simulink model "TopModel"  (R2019b)
settings: Solver=VariableStepAuto  StartTime=0.0  StopTime=10  RelTol=1e-3
model workspace (MAT data in the model file):
  J = 0.02
  Kb = 0.1
  Kf = 0.2
  Km = 0.1
  L = 0.5
  R = 2
  ctrlDen = [1 0]
  ctrlNum = [2.02136445733 8.39446937163]
settings Model: OrderedModelArguments=off  Creator=cleme  LastModifiedBy=cleme
settings DataIOCC: ReturnWorkspaceOutputs=off
settings DebuggingCC: ArithmeticOperatorsInVariantConditions=warning
settings SFSimCC: CustomCodeUndefinedFunction=UseInterfaceOnly

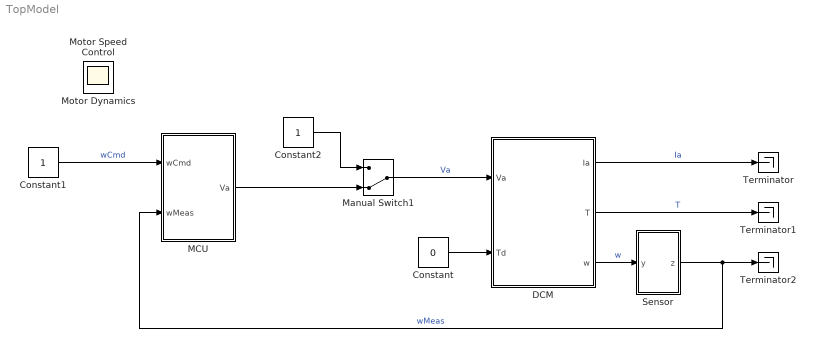
== system TopModel ==
  Constant : Constant  Value=0
  Constant1 : Constant
  Constant2 : Constant
  DCM : Subsystem
  MCU : Subsystem
  Manual Switch1 : ManualSwitch  CurrentSetting=0
  Sensor : Subsystem
  Terminator : Terminator
  Terminator1 : Terminator
  Terminator2 : Terminator
  Motor Dynamics : Scope
  Motor Speed Control : Scope
  wires:
  Constant/1 -> DCM/2(Td)
  Sensor/1(z) -> MCU/2(wMeas), Terminator2/1  "wMeas"
  DCM/3(w) -> Sensor/1(y)  "w"
  Manual Switch1/1 -> DCM/1(Va)  "Va"
  DCM/1(Ia) -> Terminator/1  "Ia"
  DCM/2(T) -> Terminator1/1  "T"
  Constant2/1 -> Manual Switch1/1
  Constant1/1 -> MCU/1(wCmd)  "wCmd"
  MCU/1(Va) -> Manual Switch1/2

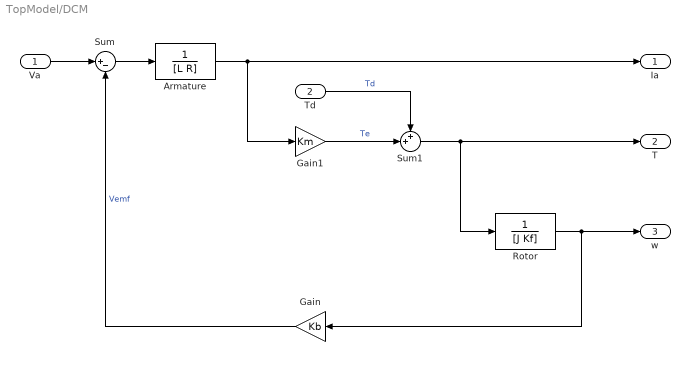
== system TopModel/DCM ==
  Va : Inport  Unit=V
  Td : Inport  Port=2  Unit=N*m
  Armature : TransferFcn  Numerator=1  Denominator=[L R]
  Gain : Gain  Gain=Kb
  Gain1 : Gain  Gain=Km
  Rotor : TransferFcn  Denominator=[J Kf]
  Sum : Sum  Inputs=|+-
  Sum1 : Sum  Inputs=++|
  Ia : Outport
  T : Outport  Port=2
  w : Outport  Port=3  Unit=rad/s  VectorParamsAs1DForOutWhenUnconnected=off
  wires:
  Sum1/1 -> Rotor/1, T/1
  Sum/1 -> Armature/1
  Va/1 -> Sum/1
  Rotor/1 -> w/1, Gain/1
  Td/1 -> Sum1/1  "Td"
  Gain/1 -> Sum/2  "Vemf"
  Armature/1 -> Ia/1, Gain1/1
  Gain1/1 -> Sum1/2  "Te"

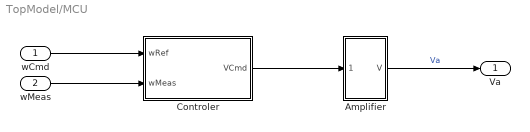
== system TopModel/MCU ==
  wCmd : Inport
  wMeas : Inport  Port=2
  Amplifier : Subsystem
  Controler : Subsystem
  Va : Outport
  wires:
  Controler/1(VCmd) -> Amplifier/1(PWM)
  wMeas/1 -> Controler/2(wMeas)
  Amplifier/1(V) -> Va/1  "Va"
  wCmd/1 -> Controler/1(wRef)

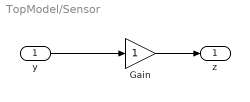
== system TopModel/Sensor ==
  y : Inport  Unit=rad/s
  Gain : Gain
  z : Outport  Unit=rad/s  VectorParamsAs1DForOutWhenUnconnected=off
  wires:
  y/1 -> Gain/1
  Gain/1 -> z/1

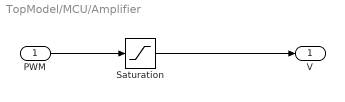
== system TopModel/MCU/Amplifier ==
  PWM : Inport  Unit=V
  Saturation : Saturate  UpperLimit=10  LowerLimit=-10
  V : Outport  Unit=V  VectorParamsAs1DForOutWhenUnconnected=off
  wires:
  PWM/1 -> Saturation/1
  Saturation/1 -> V/1

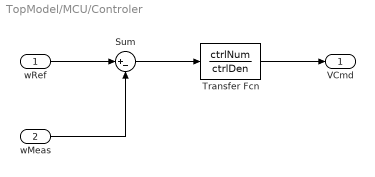
== system TopModel/MCU/Controler ==
  wRef : Inport  Unit=rad/s
  wMeas : Inport  Port=2  Unit=rad/s
  Sum : Sum  Inputs=|+-
  Transfer Fcn : TransferFcn  Numerator=ctrlNum  Denominator=ctrlDen
  VCmd : Outport  Unit=V  VectorParamsAs1DForOutWhenUnconnected=off
  wires:
  wRef/1 -> Sum/1
  wMeas/1 -> Sum/2
  Sum/1 -> Transfer Fcn/1
  Transfer Fcn/1 -> VCmd/1
